simulink model "doc_scalar_quant_2"  (R2014a)
settings: Solver=ode45  StartTime=0.0  StopTime=2*pi  RelTol=1e-3
libraries: simulink x1, commsrccod2 x1
settings Model: Creator=The MathWorks Inc.
settings DataIOCC: SignalLoggingSaveFormat=ModelDataLogs  SignalLoggingName=logsOut
settings OptimizationCC: BlockReduction=off  BooleanDataType=off  ExpressionDepthLimit=2147483647
settings DebuggingCC: SaveWithParameterizedLinksMsg=none  UnderspecifiedInitializationDetection=Classic  SignalResolutionControl=TryResolveAllWithWarning  SolverPrmCheckMsg=none  MultiTaskDSMMsg=warning  MultiTaskCondExecSysMsg=none  FcnCallInpInsideContextMsg=UseLocalSettings  StateNameClashWarn=warning  StrictBusMsg=None
settings HardwareCC: TargetUnknown=on
settings RTWCC: IncludeERTFirstTime=on
settings GRTTargetCC: TargetFcnLib=iso_c_tmw.mat  CombineOutputUpdateFcns=off  GRTInterface=on

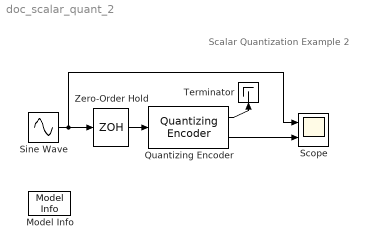
== system doc_scalar_quant_2 ==
  note: Scalar Quantization Example 2
  Model Info : simulink/Model-Wide Utilities/Model Info  InitialBlockCM=None  BlockCM=none  Frame=on  DisplayStringWithTags=Info  HorizontalTextAlignment=Center  LeftAlignmentValue=0.5  SourceBlockDiagram=doc_scalar_quant_2  TagMaxNumber=20
  Quantizing Encoder : commsrccod2/Quantizing Encoder  partition=[-1:.2:1]  codebook=[-1.1:.2:1.1]  idxDType=double
  Scope : Scope  NumInputPorts=2
      settings: YMin=-1.2~-1.2  YMax=1.2~1.2
  Sine Wave : Sin  SampleTime=0
  Terminator : Terminator
  Zero-Order Hold : ZeroOrderHold  SampleTime=.1
  wires:
  Quantizing Encoder/1 -> Terminator/1
  Quantizing Encoder/2 -> Scope/2
  Sine Wave/1 -> Scope/1, Zero-Order Hold/1
  Zero-Order Hold/1 -> Quantizing Encoder/1
